simulink model "model"  (R2021b)
settings: Solver=ode1  StartTime=0.0  StopTime=t_sim  FixedStep=st_sim  RelTol=1e-3
values from neighbouring files (symbols this model uses):
  a = 2.4    [lab3.m]    (also in lab3_2.m = 2; lab4_2.m = -2; lab4_3.m = -2; lab4_4.m = -2)
  b = 0.5    [lab3.m]    (also in lab3_2.m = 1; lab4_2.m = 5; lab4_3.m = 5; lab4_4.m = 5)
settings Model: Creator=POLUSER  LastModifiedBy=POLUSER
settings DataIOCC: SaveOutput=off  SignalLogging=off  DSMLogging=off  SaveTime=off  ReturnWorkspaceOutputs=off

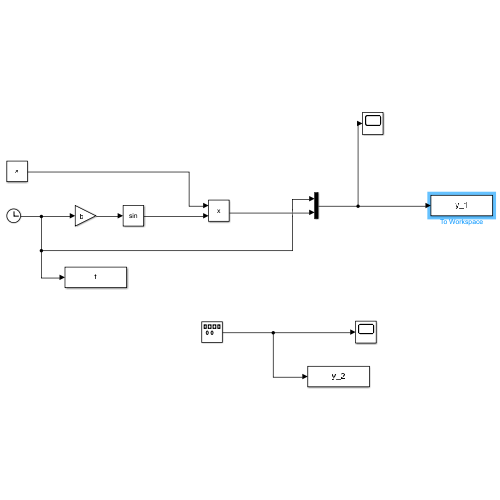
[thumbnail: Simulink's stored preview of the top-level diagram]
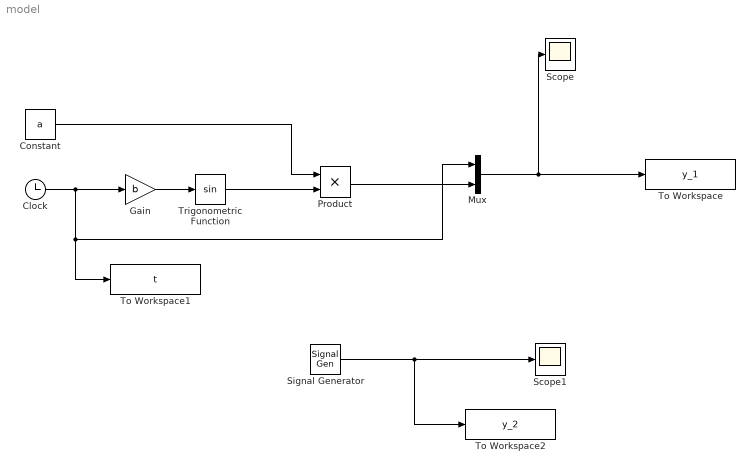
== system model ==
  Clock : Clock
  Constant : Constant  Value=a
  Gain : Gain  Gain=b
  Mux : Mux  Inputs=2
  Product : Product
  Scope : Scope
  Scope1 : Scope
  Signal Generator : SignalGenerator  Units=rad/sec
  To Workspace : ToWorkspace  VariableName=y_1  SampleTime=-1
  To Workspace1 : ToWorkspace  VariableName=t  SampleTime=-1
  To Workspace2 : ToWorkspace  VariableName=y_2  SampleTime=-1
  Trigonometric Function : Trigonometry
  wires:
  Constant/1 -> Product/1
  Gain/1 -> Trigonometric Function/1
  Clock/1 -> Gain/1, To Workspace1/1, Mux/1
  Trigonometric Function/1 -> Product/2
  Product/1 -> Mux/2
  Mux/1 -> Scope/1, To Workspace/1
  Signal Generator/1 -> Scope1/1, To Workspace2/1
